simulink model "wavelet_transform_double"  (R2024b)
settings: Solver=FixedStepDiscrete  StartTime=0.0  StopTime=100.0  RelTol=1e-3
InitFcn:
  | n=50;
  | 
  | fprintf('Size of matrix A: n = %d\n', n);
libraries: simulink x1
settings Model: DataTypeOverride=Off  Creator=valen  LastModifiedBy=valen
settings SolverCC: AlgebraicLoopSolver=TrustRegion
settings DataIOCC: LimitDataPoints=on  SaveOutput=off  SaveTime=off
settings OptimizationCC: BlockReduction=off  ConditionallyExecuteInputs=off  DefaultParameterBehavior=Inlined  LifeSpan=inf
settings DebuggingCC: AlgebraicLoopMsg=error  SingleTaskRateTransMsg=error  UnconnectedInputMsg=warning  UnconnectedOutputMsg=warning  UnconnectedLineMsg=warning  AllowSymbolicDim=off  StrictBusMsg=ErrorOnBusTreatedAsVector  SFUnexpectedBacktrackingDiag=warning  SFNoUnconditionalDefaultTransitionDiag=warning  SFExecutionAtInitializationDiag=none  ArithmeticOperatorsInVariantConditions=warning
settings HardwareCC: ProdBitPerPointer=32  ProdBitPerSizeT=32  ProdBitPerPtrDiffT=32  ProdLargestAtomicFloat=None  ProdIntDivRoundTo=Undefined  ProdEndianess=Unspecified  ProdWordSize=32  ProdHWDeviceType=ASIC/FPGA->ASIC/FPGA  ProdEqTarget=off
settings ModelReferenceCC: EnableRefExpFcnMdlSchedulingChecks=on
settings SFSimCC: SimUseLocalCustomCode=off  CustomCodeUndefinedFunction=UseInterfaceOnly
settings RTWCC: RTWUseLocalCustomCode=off  GPUComputeCapability=3.5
settings CodeAppCC: StateflowObjectComments=on
settings GRTTargetCC: TargetLangStandard=C89/C90 (ANSI)
settings ConfigComp: CovScope=ReferencedModels  CovMetricSettings=dw  CovSaveCumulativeToWorkspaceVar=on  CovSaveSingleToWorkspaceVar=on  CovExternalEMLEnable=off  CovSFcnEnable=off

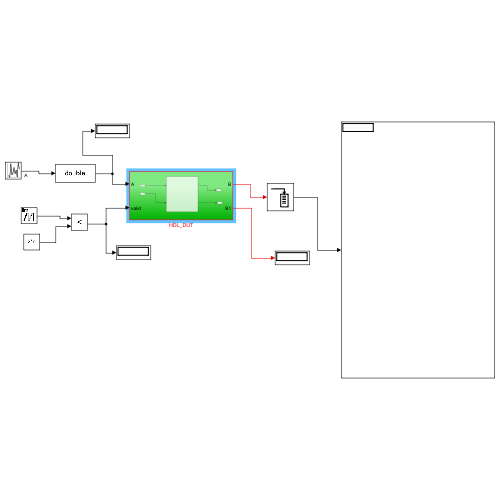
[thumbnail: Simulink's stored preview of the top-level diagram]
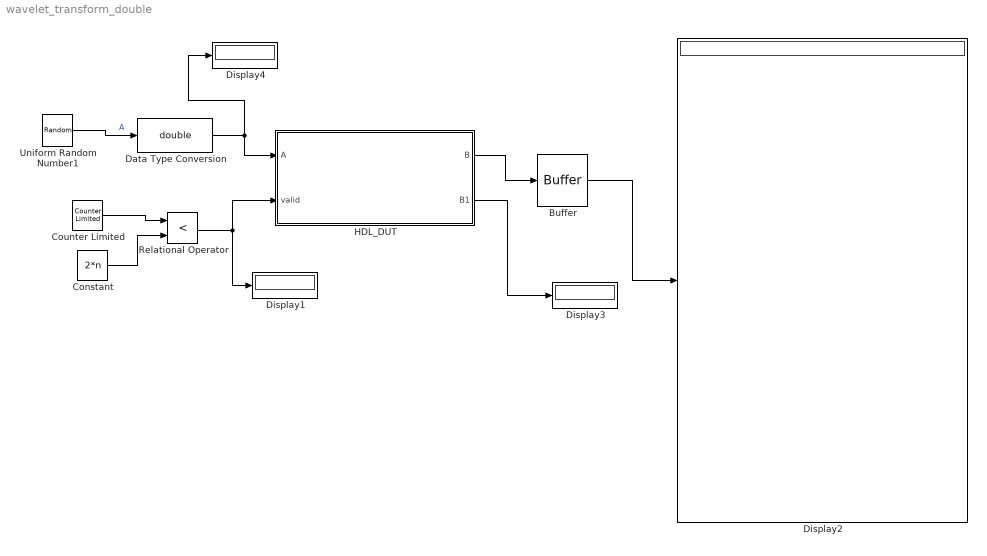
== system wavelet_transform_double ==
  Buffer : Buffer  N=100  OutputFrames=off
  Constant : Constant  Value=2*n
  Counter Limited : simulink/Sources/Counter Limited  uplimit=100  tsamp=-1
  Data Type Conversion : DataTypeConversion  OutDataTypeStr=double  SaturateOnIntegerOverflow=off  RndMeth=Floor
  Display{1..4} (4 alike) : Display
  HDL_DUT : Subsystem
  Relational Operator : RelationalOperator  Operator=<  OutDataTypeStr=boolean  RndMeth=Simplest  InputSameDT=off
  Uniform Random Number1 : UniformRandomNumber  Minimum=0  Maximum=100  Seed=n  SampleTime=10/(4*n+1)
  wires:
  Data Type Conversion/1 -> HDL_DUT/1(A), Display4/1
  Relational Operator/1 -> HDL_DUT/2(valid), Display1/1
  Counter Limited/1 -> Relational Operator/1
  Constant/1 -> Relational Operator/2
  Buffer/1 -> Display2/1
  HDL_DUT/1(B) -> Buffer/1
  Uniform Random Number1/1 -> Data Type Conversion/1  "A"
  HDL_DUT/2(B1) -> Display3/1

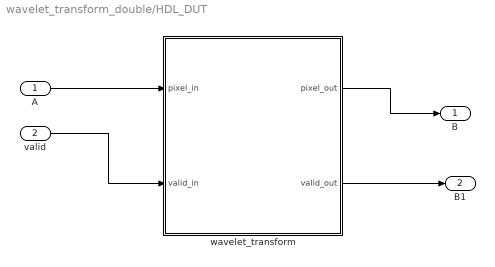
== system wavelet_transform_double/HDL_DUT ==
  A : Inport
  valid : Inport  Port=2
  wavelet_transform : MATLAB Function  TreatAsAtomicUnit=on
  B : Outport  VectorParamsAs1DForOutWhenUnconnected=off
  B1 : Outport  Port=2  VectorParamsAs1DForOutWhenUnconnected=off
  wires:
  A/1 -> wavelet_transform/1(pixel_in)
  valid/1 -> wavelet_transform/2(valid_in)
  wavelet_transform/1(pixel_out) -> B/1
  wavelet_transform/2(valid_out) -> B1/1

== matlab function wavelet_transform_double/HDL_DUT/wavelet_transform ==
  data: pixel_in input; pixel_out output; valid_in input; valid_out output
function [pixel_out,valid_out] = hardware_walevet_transform(pixel_in, valid_in)
    size = 50;
    full_size =2*size;
    LOWPASSFILTERSIZE=9;
    HIGHPASSFILTERSIZE=7;
    lowpass_filter_cpu= [0.037828455507,-0.023849465020,-0.110624404418,0.377402855613, 0.852698679009,0.377402855613, -0.110624404418,-0.023849465020, 0.037828455507];
    highpass_filter_cpu = [-0.064538882629, 0.040689417609, 0.418092273222,-0.788485616406,0.418092273222,0.040689417609,-0.064538882629];

    hi_start = int32(-floor(LOWPASSFILTERSIZE * 0.5)); % -4
    hi_end = int32(floor(LOWPASSFILTERSIZE * 0.5));  %  4
	gi_start = int32(-floor(HIGHPASSFILTERSIZE*0.5)); % -3
    gi_end = int32(floor(HIGHPASSFILTERSIZE*0.5));  %  3
    
    % Registres persistants (Hardware)
    persistent bufferA bufferhi buffergi count hi gi state;
    if isempty(state)
        bufferA = zeros(1, full_size, 'double');% RAM de stockage temporaire
        bufferhi=zeros(1, hi_end-hi_start+1, 'double');
        buffergi=zeros(1, gi_end-gi_start+1, 'double');
        count = int32(1);
        hi = hi_start;
        gi = gi_start;
        state = int32(0); % 0: Accumulation, 1: Calcul Inverse, 2: Stream Sortie
    end
    
    % Signaux de contrôle par défaut
    pixel_out = double(0);
    valid_out = double(0);
    
    switch state
        case 0 % --- Storage A ---
            if valid_in
                 % 2. Stockage dans la mémoire tampon
                bufferA(count) = double(pixel_in);     

                if count == full_size
                    count = int32(1);
                    state = int32(1); % Matrice reçue -> Passe à l'étape suivante
                else
                    count = count + 1;
                end               
            end
            
        case 1 % --- high_part ---
           x_position = (2 * count -1) + hi;
           if x_position < 1
		        %turn negative to positive
			    x_position = 1- x_position;
           elseif x_position > full_size
				x_position = full_size - (x_position - full_size);
           end    
           %now I need to restore the hi value to work with the array
		   bufferhi(hi+hi_end+1)= double(lowpass_filter_cpu(hi + hi_end+1)) * bufferA(x_position);

           if hi == hi_end
              valid_out=double(1);
              pixel_out=sum(bufferhi);
              hi = hi_start;
              
              if count == size
                count = int32(1);
                state = int32(2); % Matrice reçue -> Passe à l'étape suivante
              else
                count = count + 1;
              end
           else
              hi = hi + 1;
           end         

           

        case 2 % --- low_part ---
            x_position = (2 * count -1) + gi + 1;
            if x_position < 1
				%turn negative to positive
				x_position = 1-x_position ;
            elseif x_position >  full_size
				x_position = full_size - (x_position - full_size);
            end
            buffergi(gi+gi_end+1) = double(highpass_filter_cpu(gi + gi_end+1)) * bufferA(x_position);
		    
		                    
            if gi == gi_end
              valid_out = double(2);
              pixel_out=sum(buffergi);
              gi = gi_start;

              if count == size
                count = int32(1);
                state = int32(0); 
              else
                count = count + 1;
              end  
           else
              gi = gi + 1;
           end         

             
    end
end
